simulink model "controlGPI_pos_3dof_conMI"  (R2023b)
settings: Solver=VariableStepAuto  StartTime=0.0  StopTime=tsim  FixedStep=1e-5  MaxStep=tstep  RelTol=1e-3
undefined symbols (not defined in the file): contr_robot_params, ddq, dq, MI_Contr1, MI_Contr2, MI_Contr3, MI_motor1, MI_motor2, MI_motor3, ndof, NN_Bspline_params, NN_RBF_params, nn_select, ns, Pc, q, q0, q_cero, q_eq, robot_params, sigbuilder_block, t_qeq_init, t_tr_init, t_trtr, tau_L, tau_L_mags, tr_muestra, Wc, Zc
libraries: mcbcontrolslib x6, spsRMSLib x6, simulink x2
(part 2 of 3)

== system controlGPI_pos_3dof_conMI/Actuadores (Motores de inducción)/MI1 + PBC Torque Controller/Calculo de Potencia eléctrica ==
  u_Sab : Inport
  i_Sab : Inport  Port=2
  Demux1 : Demux  Commented=on  Outputs=3
  Demux2 : Demux  Commented=on  Outputs=3
  Demux3 : Demux  Commented=on  Outputs=3
  Demux4 : Demux  Outputs=3
  From1 : From  Commented=on  GotoTag=u_S3abc
  From2 : From  Commented=on  GotoTag=i_S3abc
  IIR Filter : mcbcontrolslib/IIR Filter  Commented=on  VariantControl=Low Pass Filter  VariantSelect=Low-pass  Filter_constant=0.04  advancedSettings=on  Ts=50e-6  cutOff_freq=132.6291
      settings: LibrarySourceBlock=mcbhdllib/Signal Management/IIR Filter
  IIR Filter1 : mcbcontrolslib/IIR Filter  Commented=on  VariantControl=Low Pass Filter  VariantSelect=Low-pass  Filter_constant=0.04  advancedSettings=on  Ts=50e-6  cutOff_freq=132.6291
      settings: LibrarySourceBlock=mcbhdllib/Signal Management/IIR Filter
  Product1 : Product
  Product2 : Product  Commented=on
  RMS : spsRMSLib/RMS  Commented=on  TrueRMS=on  Freq=60  RMSInit=120  Ts=0
  RMS1 : spsRMSLib/RMS  Commented=on  TrueRMS=on  Freq=60  RMSInit=120  Ts=0
  Scope : Scope  Commented=on
  Scope1 : Scope  Commented=on
  Scope11 : Scope  Commented=on
  Sum1 : Sum  Inputs=|+++
  Sum2 : Sum  Commented=on  Inputs=|+++
  ab0 - ABC : MATLAB Function  TreatAsAtomicUnit=on
  ab0 - ABC1 : MATLAB Function  TreatAsAtomicUnit=on
  i_S3abc1 : Scope  Commented=on  NumInputPorts=3
  u_S3abc1 : Scope  Commented=on  NumInputPorts=3
  P_elect : Outport
  u_S3abc : Outport  Port=2
  i_S3abc : Outport  Port=3
  wires:
  Sum1/1 -> P_elect/1
  Demux4/1 -> Sum1/1
  [i_S3abc] -> Product1/2
  i_Sab/1 -> ab0 - ABC1/1(BPU)
  Demux4/3 -> Sum1/3
  [u_S3abc] -> Product1/1
  Demux4/2 -> Sum1/2
  Product1/1 -> Demux4/1
  u_Sab/1 -> ab0 - ABC/1(BPU)
  [u_S3abc] -> u_S3abc/1
  [i_S3abc] -> i_S3abc/1
  ab0 - ABC/1(U) -> [u_S3abc]
  ab0 - ABC1/1(U) -> [i_S3abc]
  IIR Filter/1 -> Product2/1, Demux1/1
  RMS/1 -> Scope11/1
  Demux1/2 -> u_S3abc1/2
  Demux1/3 -> u_S3abc1/3
  Demux1/1 -> RMS/1, u_S3abc1/1
  From1/1 -> IIR Filter/1
  Demux2/1 -> RMS1/1, i_S3abc1/1
  RMS1/1 -> Scope1/1
  Demux2/2 -> i_S3abc1/2
  IIR Filter1/1 -> Product2/2, Demux2/1
  From2/1 -> IIR Filter1/1
  Demux2/3 -> i_S3abc1/3
  Demux3/2 -> Sum2/2
  Demux3/3 -> Sum2/3
  Sum2/1 -> Scope/1
  Product2/1 -> Demux3/1
  Demux3/1 -> Sum2/1

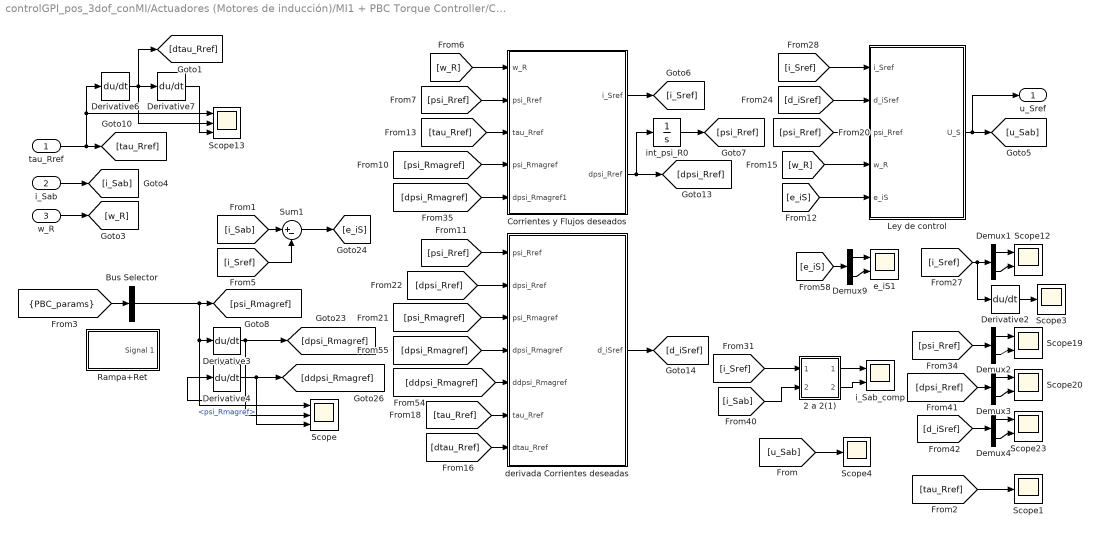
== system controlGPI_pos_3dof_conMI/Actuadores (Motores de inducción)/MI1 + PBC Torque Controller/Controlador PBC ==
  tau_Rref : Inport
  i_Sab : Inport  Port=2
  w_R : Inport  Port=3
  2 a 2(1) : Subsystem
  Bus Selector : BusSelector  OutputSignals=psi_Rmagref
  Corrientes y Flujos deseados : Subsystem
  Demux{1..4,9} (5 alike) : Demux  Outputs=2
  Derivative{2..4,6..7} (5 alike) : Derivative
  Ley de control : Subsystem
  Rampa+Ret : Subsystem  Tag=STV Subsys  LoadFcn=sigbuilder_block('load');  StartFcn=sigbuilder_block('start');  StopFcn=sigbuilder_block('stop');  ClipboardFcn=sigbuilder_block('clipboard');  mask(Sigbuilder block){tuvar=[0:10]}
      mask help: Sigbuilder GUI
      mask init:
      | if ~strcmp(get_param(bdroot(gcbh),'SimulationStatus'),'stopped') tuvar = sigbuilder_block('maskInit'); end
      settings: CopyFcn=sigbuilder_block('copy');  DeleteFcn=sigbuilder_block('delete');  ModelCloseFcn=sigbuilder_block('modelClose');  PreSaveFcn=sigbuilder_block('preSave');  PauseFcn=sigbuilder_block('pause')  ContinueFcn=sigbuilder_block('continue')  NameChangeFcn=sigbuilder_block('namechange');  OpenFcn=sigbuilder_block('open',[280.5 86.5 550.5 399.5 ]);  CloseFcn=sigbuilder_block('close');
      mask Display: plot(0, 0, 100, 100,[2, 2, 32, 32, 2], [68, 8, 8, 68, 68],[32, 2], [38, 38], [32, 19, 2],[53, 60, 44], [32, 17, 17, 2],[16, 16, 31, 31]);txt = getActiveGroup(gcbh);text(2, 100, txt,'verticalAlignment', 'top');
  Scope : Scope  NumInputPorts=3
  Scope1 : Scope
  Scope{12,19..20,23} (4 alike) : Scope  NumInputPorts=2
  Scope13 : Scope  NumInputPorts=3
  Scope3 : Scope
  Scope4 : Scope
  Sum1 : Sum  Inputs=|+-
  derivada Corrientes deseadas : Subsystem
  e_iS1 : Scope  NumInputPorts=2
  i_Sab_comp : Scope  NumInputPorts=2
  int_psi_R0 : Integrator  InitialCondition=[0.51032;0]
  u_Sref : Outport
  wires:
  Derivative3/1 -> Scope/2, Derivative4/1, [dpsi_Rmagref]
  Derivative4/1 -> [ddpsi_Rmagref], Scope/3
  Bus Selector/1 -> Scope/1, Derivative3/1, [psi_Rmagref]  "<psi_Rmagref>"
  i_Sab/1 -> [i_Sab]
  Demux1/1 -> Scope12/1
  [d_iSref] -> Demux4/1
  Demux3/2 -> Scope20/2
  Demux2/1 -> Scope19/1
  Demux1/2 -> Scope12/2
  [dpsi_Rref] -> Demux3/1
  Demux3/1 -> Scope20/1
  Demux4/1 -> Scope23/1
  [psi_Rref] -> Demux2/1
  Demux4/2 -> Scope23/2
  Demux2/2 -> Scope19/2
  [tau_Rref] -> Corrientes y Flujos deseados/3(tau_Rref)
  [w_R] -> Corrientes y Flujos deseados/1(w_R)
  int_psi_R0/1 -> [psi_Rref]
  Corrientes y Flujos deseados/2(dpsi_Rref) -> int_psi_R0/1, [dpsi_Rref]
  [psi_Rref] -> Corrientes y Flujos deseados/2(psi_Rref)
  [psi_Rmagref] -> Corrientes y Flujos deseados/4(psi_Rmagref)
  [dpsi_Rmagref] -> Corrientes y Flujos deseados/5(dpsi_Rmagref1)
  [psi_Rref] -> derivada Corrientes deseadas/1(psi_Rref)
  [dpsi_Rref] -> derivada Corrientes deseadas/2(dpsi_Rref)
  [psi_Rmagref] -> derivada Corrientes deseadas/3(psi_Rmagref)
  [dpsi_Rmagref] -> derivada Corrientes deseadas/4(dpsi_Rmagref)
  [ddpsi_Rmagref] -> derivada Corrientes deseadas/5(ddpsi_Rmagref)
  [tau_Rref] -> derivada Corrientes deseadas/6(tau_Rref)
  [dtau_Rref] -> derivada Corrientes deseadas/7(dtau_Rref)
  derivada Corrientes deseadas/1(d_iSref) -> [d_iSref]
  [e_iS] -> Demux9/1
  Demux9/1 -> e_iS1/1
  Demux9/2 -> e_iS1/2
  [i_Sab] -> Sum1/1
  [i_Sref] -> Sum1/2
  Sum1/1 -> [e_iS]
  [u_Sab] -> Scope4/1
  [i_Sref] -> Ley de control/1(i_Sref)
  [d_iSref] -> Ley de control/2(d_iSref)
  [psi_Rref] -> Ley de control/3(psi_Rref)
  [w_R] -> Ley de control/4(w_R)
  Ley de control/1(U_S) -> u_Sref/1, [u_Sab]
  [e_iS] -> Ley de control/5(e_iS)
  Derivative7/1 -> Scope13/3
  tau_Rref/1 -> Derivative6/1, Scope13/1, [tau_Rref]
  Derivative6/1 -> [dtau_Rref], Derivative7/1, Scope13/2
  2 a 2(1)/2(Out2) -> i_Sab_comp/2
  2 a 2(1)/1(Out1) -> i_Sab_comp/1
  [i_Sab] -> 2 a 2(1)/2(In2)
  [i_Sref] -> 2 a 2(1)/1(In1)
  [i_Sref] -> Derivative2/1, Demux1/1
  Derivative2/1 -> Scope3/1
  w_R/1 -> [w_R]
  [tau_Rref] -> Scope1/1
  [PBC_params] -> Bus Selector/1
  Corrientes y Flujos deseados/1(i_Sref) -> [i_Sref]

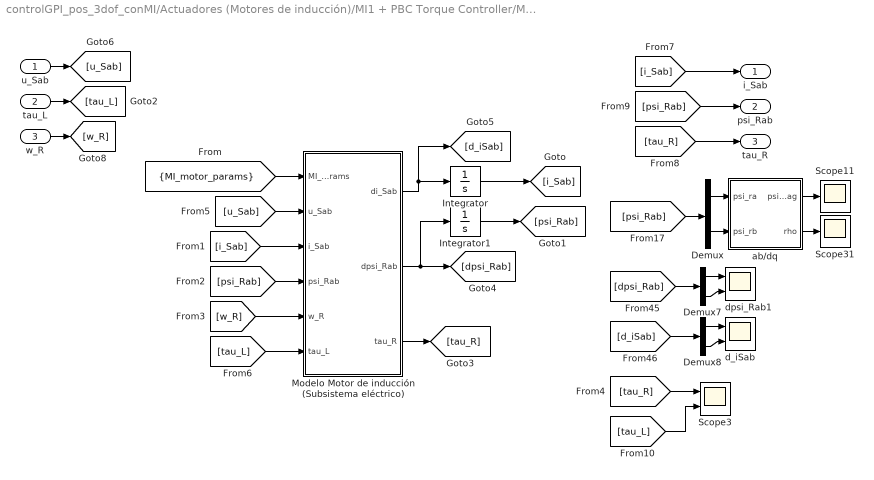
== system controlGPI_pos_3dof_conMI/Actuadores (Motores de inducción)/MI1 + PBC Torque Controller/Modelo MI (Subsistema eléctrico) ==
  u_Sab : Inport
  tau_L : Inport  Port=2
  w_R : Inport  Port=3
  Demux : Demux  Outputs=2
  Demux7 : Demux  Outputs=2
  Demux8 : Demux  Outputs=2
  Integrator : Integrator
  Integrator1 : Integrator
  Modelo Motor de inducción (Subsistema eléctrico) : MATLAB Function  TreatAsAtomicUnit=on
  Scope11 : Scope
  Scope3 : Scope  NumInputPorts=2
  Scope31 : Scope
  ab/dq : MATLAB Function  TreatAsAtomicUnit=on
  d_iSab : Scope  NumInputPorts=2
  dpsi_Rab1 : Scope  NumInputPorts=2
  i_Sab : Outport
  psi_Rab : Outport  Port=2
  tau_R : Outport  Port=3
  wires:
  Modelo Motor de inducción (Subsistema eléctrico)/1(di_Sab) -> Integrator/1, [d_iSab]
  Modelo Motor de inducción (Subsistema eléctrico)/2(dpsi_Rab) -> Integrator1/1, [dpsi_Rab]
  [w_R] -> Modelo Motor de inducción (Subsistema eléctrico)/5(w_R)
  [psi_Rab] -> Modelo Motor de inducción (Subsistema eléctrico)/4(psi_Rab)
  [i_Sab] -> Modelo Motor de inducción (Subsistema eléctrico)/3(i_Sab)
  Integrator1/1 -> [psi_Rab]
  u_Sab/1 -> [u_Sab]
  Modelo Motor de inducción (Subsistema eléctrico)/3(tau_R) -> [tau_R]
  [tau_R] -> Scope3/1
  ab/dq/1(psi_Rmag) -> Scope11/1
  [psi_Rab] -> Demux/1
  Demux7/1 -> dpsi_Rab1/1
  Demux7/2 -> dpsi_Rab1/2
  [d_iSab] -> Demux8/1
  ab/dq/2(rho) -> Scope31/1
  Demux/1 -> ab/dq/1(psi_ra)
  Demux8/2 -> d_iSab/2
  Demux8/1 -> d_iSab/1
  [dpsi_Rab] -> Demux7/1
  Demux/2 -> ab/dq/2(psi_rb)
  Integrator/1 -> [i_Sab]
  [MI_motor_params] -> Modelo Motor de inducción (Subsistema eléctrico)/1(MI_motor_params)
  [u_Sab] -> Modelo Motor de inducción (Subsistema eléctrico)/2(u_Sab)
  tau_L/1 -> [tau_L]
  [tau_L] -> Modelo Motor de inducción (Subsistema eléctrico)/6(tau_L)
  w_R/1 -> [w_R]
  [tau_R] -> tau_R/1
  [psi_Rab] -> psi_Rab/1
  [i_Sab] -> i_Sab/1
  [tau_L] -> Scope3/2

== system controlGPI_pos_3dof_conMI/Actuadores (Motores de inducción)/MI2 + PBC Torque Controller/Calculo de Potencia eléctrica ==
  u_Sab : Inport
  i_Sab : Inport  Port=2
  Demux1 : Demux  Commented=on  Outputs=3
  Demux2 : Demux  Commented=on  Outputs=3
  Demux3 : Demux  Commented=on  Outputs=3
  Demux4 : Demux  Outputs=3
  From1 : From  Commented=on  GotoTag=u_S3abc
  From2 : From  Commented=on  GotoTag=i_S3abc
  IIR Filter : mcbcontrolslib/IIR Filter  Commented=on  VariantControl=Low Pass Filter  VariantSelect=Low-pass  Filter_constant=0.04  advancedSettings=on  Ts=50e-6  cutOff_freq=132.6291
      settings: LibrarySourceBlock=mcbhdllib/Signal Management/IIR Filter
  IIR Filter1 : mcbcontrolslib/IIR Filter  Commented=on  VariantControl=Low Pass Filter  VariantSelect=Low-pass  Filter_constant=0.04  advancedSettings=on  Ts=50e-6  cutOff_freq=132.6291
      settings: LibrarySourceBlock=mcbhdllib/Signal Management/IIR Filter
  Product1 : Product
  Product2 : Product  Commented=on
  RMS : spsRMSLib/RMS  Commented=on  TrueRMS=on  Freq=60  RMSInit=120  Ts=0
  RMS1 : spsRMSLib/RMS  Commented=on  TrueRMS=on  Freq=60  RMSInit=120  Ts=0
  Scope : Scope  Commented=on
  Scope1 : Scope  Commented=on
  Scope11 : Scope  Commented=on
  Sum1 : Sum  Inputs=|+++
  Sum2 : Sum  Commented=on  Inputs=|+++
  ab0 - ABC : MATLAB Function  TreatAsAtomicUnit=on
  ab0 - ABC1 : MATLAB Function  TreatAsAtomicUnit=on
  i_S3abc1 : Scope  Commented=on  NumInputPorts=3
  u_S3abc1 : Scope  Commented=on  NumInputPorts=3
  P_elect : Outport
  u_S3abc : Outport  Port=2
  i_S3abc : Outport  Port=3
  wires:
  Sum1/1 -> P_elect/1
  Demux4/1 -> Sum1/1
  [i_S3abc] -> Product1/2
  i_Sab/1 -> ab0 - ABC1/1(BPU)
  Demux4/3 -> Sum1/3
  [u_S3abc] -> Product1/1
  Demux4/2 -> Sum1/2
  Product1/1 -> Demux4/1
  u_Sab/1 -> ab0 - ABC/1(BPU)
  [u_S3abc] -> u_S3abc/1
  [i_S3abc] -> i_S3abc/1
  ab0 - ABC/1(U) -> [u_S3abc]
  ab0 - ABC1/1(U) -> [i_S3abc]
  IIR Filter/1 -> Product2/1, Demux1/1
  RMS/1 -> Scope11/1
  Demux1/2 -> u_S3abc1/2
  Demux1/3 -> u_S3abc1/3
  Demux1/1 -> RMS/1, u_S3abc1/1
  From1/1 -> IIR Filter/1
  Demux2/1 -> RMS1/1, i_S3abc1/1
  RMS1/1 -> Scope1/1
  Demux2/2 -> i_S3abc1/2
  IIR Filter1/1 -> Product2/2, Demux2/1
  From2/1 -> IIR Filter1/1
  Demux2/3 -> i_S3abc1/3
  Demux3/2 -> Sum2/2
  Demux3/3 -> Sum2/3
  Sum2/1 -> Scope/1
  Product2/1 -> Demux3/1
  Demux3/1 -> Sum2/1

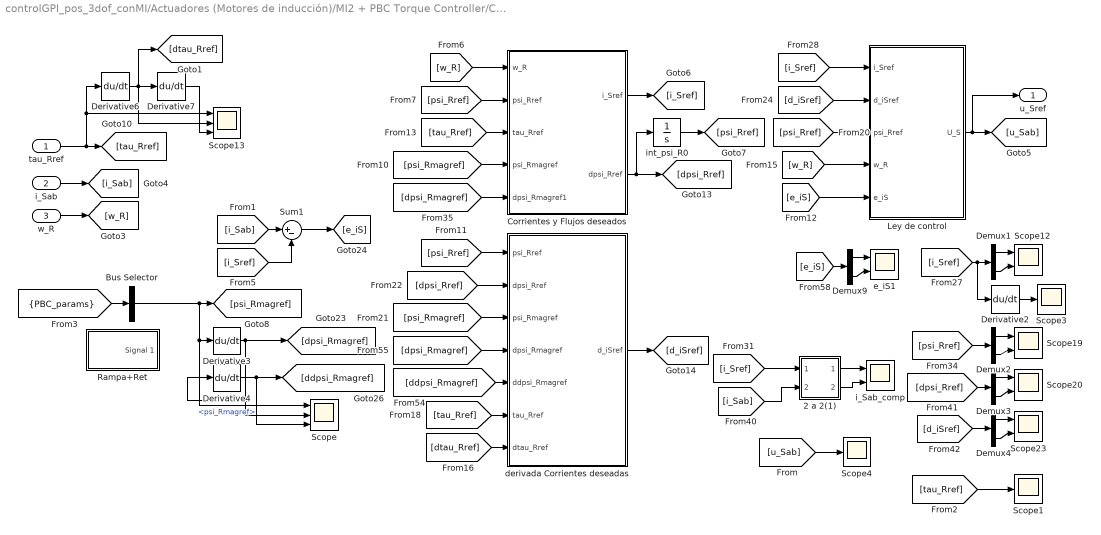
== system controlGPI_pos_3dof_conMI/Actuadores (Motores de inducción)/MI2 + PBC Torque Controller/Controlador PBC ==
  tau_Rref : Inport
  i_Sab : Inport  Port=2
  w_R : Inport  Port=3
  2 a 2(1) : Subsystem
  Bus Selector : BusSelector  OutputSignals=psi_Rmagref
  Corrientes y Flujos deseados : Subsystem
  Demux{1..4,9} (5 alike) : Demux  Outputs=2
  Derivative{2..4,6..7} (5 alike) : Derivative
  Ley de control : Subsystem
  Rampa+Ret : Subsystem  Tag=STV Subsys  LoadFcn=sigbuilder_block('load');  StartFcn=sigbuilder_block('start');  StopFcn=sigbuilder_block('stop');  ClipboardFcn=sigbuilder_block('clipboard');  mask(Sigbuilder block){tuvar=[0:10]}
      mask help: Sigbuilder GUI
      mask init:
      | if ~strcmp(get_param(bdroot(gcbh),'SimulationStatus'),'stopped') tuvar = sigbuilder_block('maskInit'); end
      settings: CopyFcn=sigbuilder_block('copy');  DeleteFcn=sigbuilder_block('delete');  ModelCloseFcn=sigbuilder_block('modelClose');  PreSaveFcn=sigbuilder_block('preSave');  PauseFcn=sigbuilder_block('pause')  ContinueFcn=sigbuilder_block('continue')  NameChangeFcn=sigbuilder_block('namechange');  OpenFcn=sigbuilder_block('open',[280.5 86.5 550.5 399.5 ]);  CloseFcn=sigbuilder_block('close');
      mask Display: plot(0, 0, 100, 100,[2, 2, 32, 32, 2], [68, 8, 8, 68, 68],[32, 2], [38, 38], [32, 19, 2],[53, 60, 44], [32, 17, 17, 2],[16, 16, 31, 31]);txt = getActiveGroup(gcbh);text(2, 100, txt,'verticalAlignment', 'top');
  Scope : Scope  NumInputPorts=3
  Scope1 : Scope
  Scope{12,19..20,23} (4 alike) : Scope  NumInputPorts=2
  Scope13 : Scope  NumInputPorts=3
  Scope3 : Scope
  Scope4 : Scope
  Sum1 : Sum  Inputs=|+-
  derivada Corrientes deseadas : Subsystem
  e_iS1 : Scope  NumInputPorts=2
  i_Sab_comp : Scope  NumInputPorts=2
  int_psi_R0 : Integrator  InitialCondition=[0.51032;0]
  u_Sref : Outport
  wires:
  Derivative3/1 -> Scope/2, Derivative4/1, [dpsi_Rmagref]
  Derivative4/1 -> [ddpsi_Rmagref], Scope/3
  Bus Selector/1 -> Scope/1, Derivative3/1, [psi_Rmagref]  "<psi_Rmagref>"
  i_Sab/1 -> [i_Sab]
  Demux1/1 -> Scope12/1
  [d_iSref] -> Demux4/1
  Demux3/2 -> Scope20/2
  Demux2/1 -> Scope19/1
  Demux1/2 -> Scope12/2
  [dpsi_Rref] -> Demux3/1
  Demux3/1 -> Scope20/1
  Demux4/1 -> Scope23/1
  [psi_Rref] -> Demux2/1
  Demux4/2 -> Scope23/2
  Demux2/2 -> Scope19/2
  [tau_Rref] -> Corrientes y Flujos deseados/3(tau_Rref)
  [w_R] -> Corrientes y Flujos deseados/1(w_R)
  int_psi_R0/1 -> [psi_Rref]
  Corrientes y Flujos deseados/2(dpsi_Rref) -> int_psi_R0/1, [dpsi_Rref]
  [psi_Rref] -> Corrientes y Flujos deseados/2(psi_Rref)
  [psi_Rmagref] -> Corrientes y Flujos deseados/4(psi_Rmagref)
  [dpsi_Rmagref] -> Corrientes y Flujos deseados/5(dpsi_Rmagref1)
  [psi_Rref] -> derivada Corrientes deseadas/1(psi_Rref)
  [dpsi_Rref] -> derivada Corrientes deseadas/2(dpsi_Rref)
  [psi_Rmagref] -> derivada Corrientes deseadas/3(psi_Rmagref)
  [dpsi_Rmagref] -> derivada Corrientes deseadas/4(dpsi_Rmagref)
  [ddpsi_Rmagref] -> derivada Corrientes deseadas/5(ddpsi_Rmagref)
  [tau_Rref] -> derivada Corrientes deseadas/6(tau_Rref)
  [dtau_Rref] -> derivada Corrientes deseadas/7(dtau_Rref)
  derivada Corrientes deseadas/1(d_iSref) -> [d_iSref]
  [e_iS] -> Demux9/1
  Demux9/1 -> e_iS1/1
  Demux9/2 -> e_iS1/2
  [i_Sab] -> Sum1/1
  [i_Sref] -> Sum1/2
  Sum1/1 -> [e_iS]
  [u_Sab] -> Scope4/1
  [i_Sref] -> Ley de control/1(i_Sref)
  [d_iSref] -> Ley de control/2(d_iSref)
  [psi_Rref] -> Ley de control/3(psi_Rref)
  [w_R] -> Ley de control/4(w_R)
  Ley de control/1(U_S) -> u_Sref/1, [u_Sab]
  [e_iS] -> Ley de control/5(e_iS)
  Derivative7/1 -> Scope13/3
  tau_Rref/1 -> Derivative6/1, Scope13/1, [tau_Rref]
  Derivative6/1 -> [dtau_Rref], Derivative7/1, Scope13/2
  2 a 2(1)/2(Out2) -> i_Sab_comp/2
  2 a 2(1)/1(Out1) -> i_Sab_comp/1
  [i_Sab] -> 2 a 2(1)/2(In2)
  [i_Sref] -> 2 a 2(1)/1(In1)
  [i_Sref] -> Derivative2/1, Demux1/1
  Derivative2/1 -> Scope3/1
  w_R/1 -> [w_R]
  [tau_Rref] -> Scope1/1
  [PBC_params] -> Bus Selector/1
  Corrientes y Flujos deseados/1(i_Sref) -> [i_Sref]

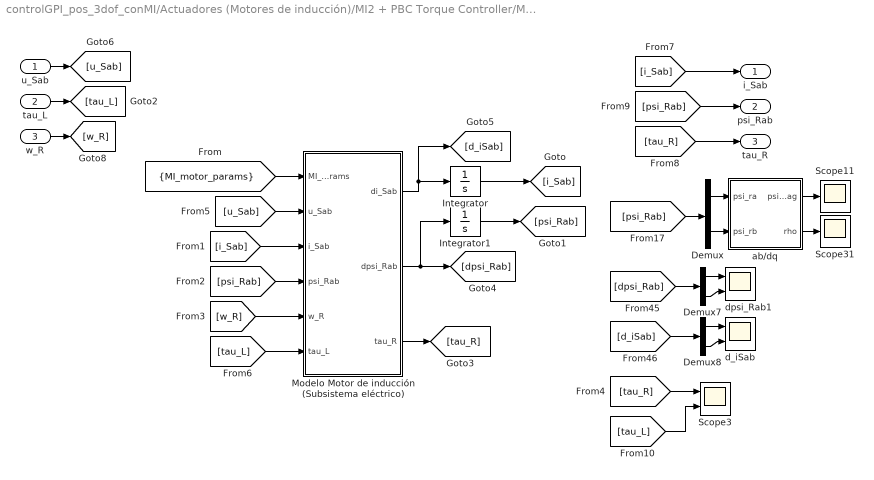
== system controlGPI_pos_3dof_conMI/Actuadores (Motores de inducción)/MI2 + PBC Torque Controller/Modelo MI (Subsistema eléctrico) ==
  u_Sab : Inport
  tau_L : Inport  Port=2
  w_R : Inport  Port=3
  Demux : Demux  Outputs=2
  Demux7 : Demux  Outputs=2
  Demux8 : Demux  Outputs=2
  Integrator : Integrator
  Integrator1 : Integrator
  Modelo Motor de inducción (Subsistema eléctrico) : MATLAB Function  TreatAsAtomicUnit=on
  Scope11 : Scope
  Scope3 : Scope  NumInputPorts=2
  Scope31 : Scope
  ab/dq : MATLAB Function  TreatAsAtomicUnit=on
  d_iSab : Scope  NumInputPorts=2
  dpsi_Rab1 : Scope  NumInputPorts=2
  i_Sab : Outport
  psi_Rab : Outport  Port=2
  tau_R : Outport  Port=3
  wires:
  Modelo Motor de inducción (Subsistema eléctrico)/1(di_Sab) -> Integrator/1, [d_iSab]
  Modelo Motor de inducción (Subsistema eléctrico)/2(dpsi_Rab) -> Integrator1/1, [dpsi_Rab]
  [w_R] -> Modelo Motor de inducción (Subsistema eléctrico)/5(w_R)
  [psi_Rab] -> Modelo Motor de inducción (Subsistema eléctrico)/4(psi_Rab)
  [i_Sab] -> Modelo Motor de inducción (Subsistema eléctrico)/3(i_Sab)
  Integrator1/1 -> [psi_Rab]
  u_Sab/1 -> [u_Sab]
  Modelo Motor de inducción (Subsistema eléctrico)/3(tau_R) -> [tau_R]
  [tau_R] -> Scope3/1
  ab/dq/1(psi_Rmag) -> Scope11/1
  [psi_Rab] -> Demux/1
  Demux7/1 -> dpsi_Rab1/1
  Demux7/2 -> dpsi_Rab1/2
  [d_iSab] -> Demux8/1
  ab/dq/2(rho) -> Scope31/1
  Demux/1 -> ab/dq/1(psi_ra)
  Demux8/2 -> d_iSab/2
  Demux8/1 -> d_iSab/1
  [dpsi_Rab] -> Demux7/1
  Demux/2 -> ab/dq/2(psi_rb)
  Integrator/1 -> [i_Sab]
  [MI_motor_params] -> Modelo Motor de inducción (Subsistema eléctrico)/1(MI_motor_params)
  [u_Sab] -> Modelo Motor de inducción (Subsistema eléctrico)/2(u_Sab)
  tau_L/1 -> [tau_L]
  [tau_L] -> Modelo Motor de inducción (Subsistema eléctrico)/6(tau_L)
  w_R/1 -> [w_R]
  [tau_R] -> tau_R/1
  [psi_Rab] -> psi_Rab/1
  [i_Sab] -> i_Sab/1
  [tau_L] -> Scope3/2

== system controlGPI_pos_3dof_conMI/Actuadores (Motores de inducción)/MI3 + PBC Torque Controller/Calculo de Potencia eléctrica ==
  u_Sab : Inport
  i_Sab : Inport  Port=2
  Demux1 : Demux  Commented=on  Outputs=3
  Demux2 : Demux  Commented=on  Outputs=3
  Demux3 : Demux  Commented=on  Outputs=3
  Demux4 : Demux  Outputs=3
  From1 : From  Commented=on  GotoTag=u_S3abc
  From2 : From  Commented=on  GotoTag=i_S3abc
  IIR Filter : mcbcontrolslib/IIR Filter  Commented=on  VariantControl=Low Pass Filter  VariantSelect=Low-pass  Filter_constant=0.04  advancedSettings=on  Ts=50e-6  cutOff_freq=132.6291
      settings: LibrarySourceBlock=mcbhdllib/Signal Management/IIR Filter
  IIR Filter1 : mcbcontrolslib/IIR Filter  Commented=on  VariantControl=Low Pass Filter  VariantSelect=Low-pass  Filter_constant=0.04  advancedSettings=on  Ts=50e-6  cutOff_freq=132.6291
      settings: LibrarySourceBlock=mcbhdllib/Signal Management/IIR Filter
  Product1 : Product
  Product2 : Product  Commented=on
  RMS : spsRMSLib/RMS  Commented=on  TrueRMS=on  Freq=60  RMSInit=120  Ts=0
  RMS1 : spsRMSLib/RMS  Commented=on  TrueRMS=on  Freq=60  RMSInit=120  Ts=0
  Scope : Scope  Commented=on
  Scope1 : Scope  Commented=on
  Scope11 : Scope  Commented=on
  Sum1 : Sum  Inputs=|+++
  Sum2 : Sum  Commented=on  Inputs=|+++
  ab0 - ABC : MATLAB Function  TreatAsAtomicUnit=on
  ab0 - ABC1 : MATLAB Function  TreatAsAtomicUnit=on
  i_S3abc1 : Scope  Commented=on  NumInputPorts=3
  u_S3abc1 : Scope  Commented=on  NumInputPorts=3
  P_elect : Outport
  u_S3abc : Outport  Port=2
  i_S3abc : Outport  Port=3
  wires:
  Sum1/1 -> P_elect/1
  Demux4/1 -> Sum1/1
  [i_S3abc] -> Product1/2
  i_Sab/1 -> ab0 - ABC1/1(BPU)
  Demux4/3 -> Sum1/3
  [u_S3abc] -> Product1/1
  Demux4/2 -> Sum1/2
  Product1/1 -> Demux4/1
  u_Sab/1 -> ab0 - ABC/1(BPU)
  [u_S3abc] -> u_S3abc/1
  [i_S3abc] -> i_S3abc/1
  ab0 - ABC/1(U) -> [u_S3abc]
  ab0 - ABC1/1(U) -> [i_S3abc]
  IIR Filter/1 -> Product2/1, Demux1/1
  RMS/1 -> Scope11/1
  Demux1/2 -> u_S3abc1/2
  Demux1/3 -> u_S3abc1/3
  Demux1/1 -> RMS/1, u_S3abc1/1
  From1/1 -> IIR Filter/1
  Demux2/1 -> RMS1/1, i_S3abc1/1
  RMS1/1 -> Scope1/1
  Demux2/2 -> i_S3abc1/2
  IIR Filter1/1 -> Product2/2, Demux2/1
  From2/1 -> IIR Filter1/1
  Demux2/3 -> i_S3abc1/3
  Demux3/2 -> Sum2/2
  Demux3/3 -> Sum2/3
  Sum2/1 -> Scope/1
  Product2/1 -> Demux3/1
  Demux3/1 -> Sum2/1

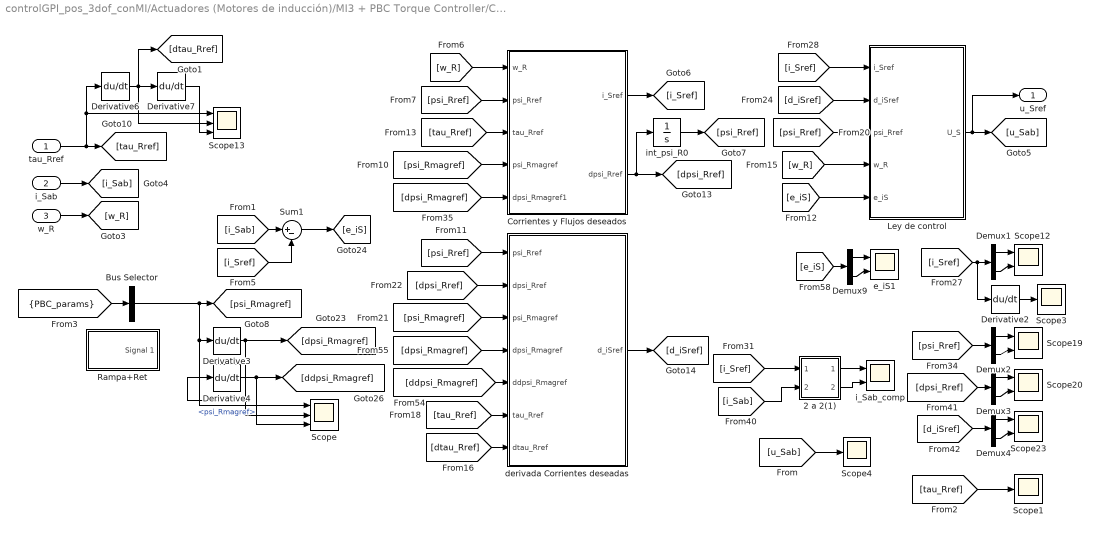
== system controlGPI_pos_3dof_conMI/Actuadores (Motores de inducción)/MI3 + PBC Torque Controller/Controlador PBC ==
  tau_Rref : Inport
  i_Sab : Inport  Port=2
  w_R : Inport  Port=3
  2 a 2(1) : Subsystem
  Bus Selector : BusSelector  OutputSignals=psi_Rmagref
  Corrientes y Flujos deseados : Subsystem
  Demux{1..4,9} (5 alike) : Demux  Outputs=2
  Derivative{2..4,6..7} (5 alike) : Derivative
  Ley de control : Subsystem
  Rampa+Ret : Subsystem  Tag=STV Subsys  LoadFcn=sigbuilder_block('load');  StartFcn=sigbuilder_block('start');  StopFcn=sigbuilder_block('stop');  ClipboardFcn=sigbuilder_block('clipboard');  mask(Sigbuilder block){tuvar=[0:10]}
      mask help: Sigbuilder GUI
      mask init:
      | if ~strcmp(get_param(bdroot(gcbh),'SimulationStatus'),'stopped') tuvar = sigbuilder_block('maskInit'); end
      settings: CopyFcn=sigbuilder_block('copy');  DeleteFcn=sigbuilder_block('delete');  ModelCloseFcn=sigbuilder_block('modelClose');  PreSaveFcn=sigbuilder_block('preSave');  PauseFcn=sigbuilder_block('pause')  ContinueFcn=sigbuilder_block('continue')  NameChangeFcn=sigbuilder_block('namechange');  OpenFcn=sigbuilder_block('open',[280.5 86.5 550.5 399.5 ]);  CloseFcn=sigbuilder_block('close');
      mask Display: plot(0, 0, 100, 100,[2, 2, 32, 32, 2], [68, 8, 8, 68, 68],[32, 2], [38, 38], [32, 19, 2],[53, 60, 44], [32, 17, 17, 2],[16, 16, 31, 31]);txt = getActiveGroup(gcbh);text(2, 100, txt,'verticalAlignment', 'top');
  Scope : Scope  NumInputPorts=3
  Scope1 : Scope
  Scope{12,19..20,23} (4 alike) : Scope  NumInputPorts=2
  Scope13 : Scope  NumInputPorts=3
  Scope3 : Scope
  Scope4 : Scope
  Sum1 : Sum  Inputs=|+-
  derivada Corrientes deseadas : Subsystem
  e_iS1 : Scope  NumInputPorts=2
  i_Sab_comp : Scope  NumInputPorts=2
  int_psi_R0 : Integrator  InitialCondition=[0.51032;0]
  u_Sref : Outport
  wires:
  Derivative3/1 -> Scope/2, Derivative4/1, [dpsi_Rmagref]
  Derivative4/1 -> [ddpsi_Rmagref], Scope/3
  Bus Selector/1 -> Scope/1, Derivative3/1, [psi_Rmagref]  "<psi_Rmagref>"
  i_Sab/1 -> [i_Sab]
  Demux1/1 -> Scope12/1
  [d_iSref] -> Demux4/1
  Demux3/2 -> Scope20/2
  Demux2/1 -> Scope19/1
  Demux1/2 -> Scope12/2
  [dpsi_Rref] -> Demux3/1
  Demux3/1 -> Scope20/1
  Demux4/1 -> Scope23/1
  [psi_Rref] -> Demux2/1
  Demux4/2 -> Scope23/2
  Demux2/2 -> Scope19/2
  [tau_Rref] -> Corrientes y Flujos deseados/3(tau_Rref)
  [w_R] -> Corrientes y Flujos deseados/1(w_R)
  int_psi_R0/1 -> [psi_Rref]
  Corrientes y Flujos deseados/2(dpsi_Rref) -> int_psi_R0/1, [dpsi_Rref]
  [psi_Rref] -> Corrientes y Flujos deseados/2(psi_Rref)
  [psi_Rmagref] -> Corrientes y Flujos deseados/4(psi_Rmagref)
  [dpsi_Rmagref] -> Corrientes y Flujos deseados/5(dpsi_Rmagref1)
  [psi_Rref] -> derivada Corrientes deseadas/1(psi_Rref)
  [dpsi_Rref] -> derivada Corrientes deseadas/2(dpsi_Rref)
  [psi_Rmagref] -> derivada Corrientes deseadas/3(psi_Rmagref)
  [dpsi_Rmagref] -> derivada Corrientes deseadas/4(dpsi_Rmagref)
  [ddpsi_Rmagref] -> derivada Corrientes deseadas/5(ddpsi_Rmagref)
  [tau_Rref] -> derivada Corrientes deseadas/6(tau_Rref)
  [dtau_Rref] -> derivada Corrientes deseadas/7(dtau_Rref)
  derivada Corrientes deseadas/1(d_iSref) -> [d_iSref]
  [e_iS] -> Demux9/1
  Demux9/1 -> e_iS1/1
  Demux9/2 -> e_iS1/2
  [i_Sab] -> Sum1/1
  [i_Sref] -> Sum1/2
  Sum1/1 -> [e_iS]
  [u_Sab] -> Scope4/1
  [i_Sref] -> Ley de control/1(i_Sref)
  [d_iSref] -> Ley de control/2(d_iSref)
  [psi_Rref] -> Ley de control/3(psi_Rref)
  [w_R] -> Ley de control/4(w_R)
  Ley de control/1(U_S) -> u_Sref/1, [u_Sab]
  [e_iS] -> Ley de control/5(e_iS)
  Derivative7/1 -> Scope13/3
  tau_Rref/1 -> Derivative6/1, Scope13/1, [tau_Rref]
  Derivative6/1 -> [dtau_Rref], Derivative7/1, Scope13/2
  2 a 2(1)/2(Out2) -> i_Sab_comp/2
  2 a 2(1)/1(Out1) -> i_Sab_comp/1
  [i_Sab] -> 2 a 2(1)/2(In2)
  [i_Sref] -> 2 a 2(1)/1(In1)
  [i_Sref] -> Derivative2/1, Demux1/1
  Derivative2/1 -> Scope3/1
  w_R/1 -> [w_R]
  [tau_Rref] -> Scope1/1
  [PBC_params] -> Bus Selector/1
  Corrientes y Flujos deseados/1(i_Sref) -> [i_Sref]

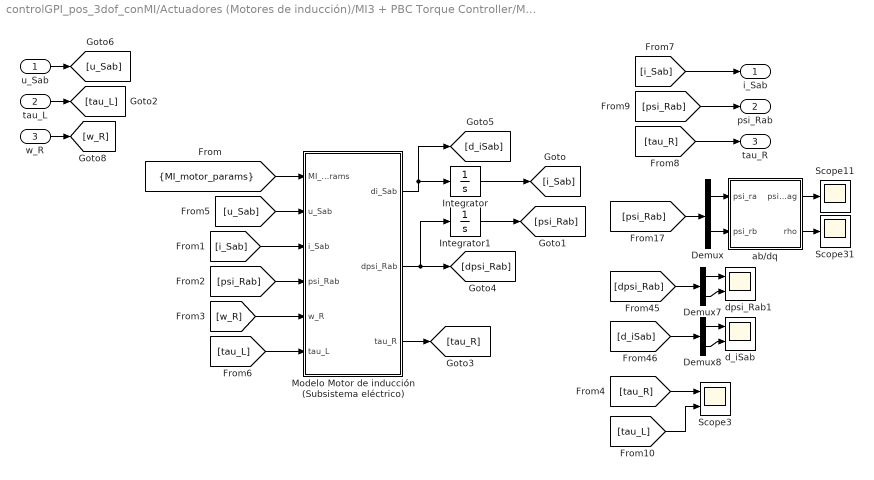
== system controlGPI_pos_3dof_conMI/Actuadores (Motores de inducción)/MI3 + PBC Torque Controller/Modelo MI (Subsistema eléctrico) ==
  u_Sab : Inport
  tau_L : Inport  Port=2
  w_R : Inport  Port=3
  Demux : Demux  Outputs=2
  Demux7 : Demux  Outputs=2
  Demux8 : Demux  Outputs=2
  Integrator : Integrator
  Integrator1 : Integrator
  Modelo Motor de inducción (Subsistema eléctrico) : MATLAB Function  TreatAsAtomicUnit=on
  Scope11 : Scope
  Scope3 : Scope  NumInputPorts=2
  Scope31 : Scope
  ab/dq : MATLAB Function  TreatAsAtomicUnit=on
  d_iSab : Scope  NumInputPorts=2
  dpsi_Rab1 : Scope  NumInputPorts=2
  i_Sab : Outport
  psi_Rab : Outport  Port=2
  tau_R : Outport  Port=3
  wires:
  Modelo Motor de inducción (Subsistema eléctrico)/1(di_Sab) -> Integrator/1, [d_iSab]
  Modelo Motor de inducción (Subsistema eléctrico)/2(dpsi_Rab) -> Integrator1/1, [dpsi_Rab]
  [w_R] -> Modelo Motor de inducción (Subsistema eléctrico)/5(w_R)
  [psi_Rab] -> Modelo Motor de inducción (Subsistema eléctrico)/4(psi_Rab)
  [i_Sab] -> Modelo Motor de inducción (Subsistema eléctrico)/3(i_Sab)
  Integrator1/1 -> [psi_Rab]
  u_Sab/1 -> [u_Sab]
  Modelo Motor de inducción (Subsistema eléctrico)/3(tau_R) -> [tau_R]
  [tau_R] -> Scope3/1
  ab/dq/1(psi_Rmag) -> Scope11/1
  [psi_Rab] -> Demux/1
  Demux7/1 -> dpsi_Rab1/1
  Demux7/2 -> dpsi_Rab1/2
  [d_iSab] -> Demux8/1
  ab/dq/2(rho) -> Scope31/1
  Demux/1 -> ab/dq/1(psi_ra)
  Demux8/2 -> d_iSab/2
  Demux8/1 -> d_iSab/1
  [dpsi_Rab] -> Demux7/1
  Demux/2 -> ab/dq/2(psi_rb)
  Integrator/1 -> [i_Sab]
  [MI_motor_params] -> Modelo Motor de inducción (Subsistema eléctrico)/1(MI_motor_params)
  [u_Sab] -> Modelo Motor de inducción (Subsistema eléctrico)/2(u_Sab)
  tau_L/1 -> [tau_L]
  [tau_L] -> Modelo Motor de inducción (Subsistema eléctrico)/6(tau_L)
  w_R/1 -> [w_R]
  [tau_R] -> tau_R/1
  [psi_Rab] -> psi_Rab/1
  [i_Sab] -> i_Sab/1
  [tau_L] -> Scope3/2

== system controlGPI_pos_3dof_conMI/ControladorGPI + NN/Red neuronal/B-Spline NNs ==
  e_q : Inport
  de_q : Inport  Port=2
  e_p : Inport  Port=3
  Action Port : ActionPort  ActionPortLabel=if(u1 == 1)
  Bus Creator : BusCreator  Inputs=3
  Constant3 : Constant  Value=NN_Bspline_params.struct  OutDataTypeStr=Bus: NN_Bspline_params_bus
  Data Store Memory : DataStoreMemory  DataStoreName=weightsWc  WriteAfterWriteMsg=warning  InitialValue=NN_Bspline_params.weights.weightWc  ShowAdditionalParam=off  OutDataTypeStr=double
  Data Store Memory1 : DataStoreMemory  DataStoreName=weightsZc  WriteAfterWriteMsg=warning  InitialValue=NN_Bspline_params.weights.weightZc  ShowAdditionalParam=off  OutDataTypeStr=double
  Data Store Memory2 : DataStoreMemory  DataStoreName=weightsPc  WriteAfterWriteMsg=warning  InitialValue=NN_Bspline_params.weights.weightPc  ShowAdditionalParam=off  OutDataTypeStr=double
  Data Store Read : DataStoreRead  DataStoreName=weightsPc  IndexOptions=Index vector (dialog)  Indices=1  OutputSizes=1
  Data Store Read1 : DataStoreRead  DataStoreName=weightsWc  IndexOptions=Index vector (dialog)  Indices=1  OutputSizes=1
  Data Store Read2 : DataStoreRead  DataStoreName=weightsZc  IndexOptions=Index vector (dialog)  Indices=1  OutputSizes=1
  Data Store Read3 : DataStoreRead  DataStoreName=weightsWc  IndexOptions=Index vector (dialog)  Indices=1  OutputSizes=1
  Data Store Read4 : DataStoreRead  DataStoreName=weightsZc  IndexOptions=Index vector (dialog)  Indices=1  OutputSizes=1
  Data Store Read5 : DataStoreRead  DataStoreName=weightsPc  IndexOptions=Index vector (dialog)  Indices=1  OutputSizes=1
  Data Store Read6 : DataStoreRead  DataStoreName=weightsWc  IndexOptions=Index vector (dialog)  Indices=1  OutputSizes=1
  Data Store Read7 : DataStoreRead  DataStoreName=weightsZc  IndexOptions=Index vector (dialog)  Indices=1  OutputSizes=1
  Data Store Read8 : DataStoreRead  DataStoreName=weightsPc  IndexOptions=Index vector (dialog)  Indices=1  OutputSizes=1
  Data Store Write : DataStoreWrite  DataStoreName=weightsPc  IndexOptions=Index vector (dialog)  Indices=1  OutputSizes=1
  Data Store Write1 : DataStoreWrite  DataStoreName=weightsZc  IndexOptions=Index vector (dialog)  Indices=1  OutputSizes=1
  Data Store Write2 : DataStoreWrite  DataStoreName=weightsWc  IndexOptions=Index vector (dialog)  Indices=1  OutputSizes=1
  Demux : Demux  Outputs=3
  Mux : Mux  Inputs=3
  Mux1 : Mux  Inputs=3
  Mux2 : Mux  Inputs=3
  Red Neuronal B-spline : MATLAB Function  TreatAsAtomicUnit=on
  To Workspace : ToWorkspace  VariableName=BSplineNN_weights  SaveFormat=Timeseries  SampleTime=-1
  bspline_gpi_params : Scope  NumInputPorts=3
  weights_BSplineNN : Scope  NumInputPorts=3
  Wc : Outport
  Zc : Outport  Port=2
  Pc : Outport  Port=3
  wires:
  e_q/1 -> Red Neuronal B-spline/2(e_q)
  [Bspline_params] -> Red Neuronal B-spline/1(NN_Bspline_params)
  Red Neuronal B-spline/1(Wc) -> bspline_gpi_params/1, Wc/1
  Red Neuronal B-spline/2(Zc) -> bspline_gpi_params/2, Zc/1
  Red Neuronal B-spline/3(Pc) -> bspline_gpi_params/3, Pc/1
  Constant3/1 -> [Bspline_params]
  Data Store Read1/1 -> Bus Creator/1  "weightsWc"
  Data Store Read5/1 -> Bus Creator/3  "weightsPc"
  Bus Creator/1 -> To Workspace/1
  Data Store Read4/1 -> Bus Creator/2  "weightsZc"
  Red Neuronal B-spline/4(newweightsWc) -> Data Store Write2/1
  Red Neuronal B-spline/5(newweightsZc) -> Data Store Write1/1
  Red Neuronal B-spline/6(newweightsPc) -> Data Store Write/1
  Data Store Read3/1 -> Red Neuronal B-spline/6(weightsWc)
  Data Store Read2/1 -> Red Neuronal B-spline/7(weightsZc)
  Data Store Read/1 -> Red Neuronal B-spline/8(weightsPc)
  Data Store Read6/1 -> weights_BSplineNN/1  "weightsWc"
  Data Store Read7/1 -> weights_BSplineNN/2  "weightsZc"
  Data Store Read8/1 -> weights_BSplineNN/3  "weightsPc"
  Mux1/1 -> Red Neuronal B-spline/4(e_py)
  Mux2/1 -> Red Neuronal B-spline/5(e_pz)
  Demux/3 -> Mux2/3, Mux2/2, Mux2/1
  e_p/1 -> Demux/1
  Demux/1 -> Mux/3, Mux/1, Mux/2
  Mux/1 -> Red Neuronal B-spline/3(e_px)
  Demux/2 -> Mux1/1, Mux1/3, Mux1/2

== system controlGPI_pos_3dof_conMI/ControladorGPI + NN/Red neuronal/Constants ==
  Action Port : ActionPort  ActionPortLabel=else
  Constant : Constant  Value=Wc
  Constant1 : Constant  Value=Zc
  Constant2 : Constant  Value=Pc
  Scope1 : Scope  NumInputPorts=3
  Wc : Outport
  Zc : Outport  Port=2
  Pc : Outport  Port=3
  wires:
  Constant/1 -> Wc/1, Scope1/1
  Constant2/1 -> Scope1/3, Pc/1
  Constant1/1 -> Zc/1, Scope1/2

== system controlGPI_pos_3dof_conMI/ControladorGPI + NN/Red neuronal/RBF NNs ==
  e_q : Inport
  de_q : Inport  Port=2
  e_p : Inport  Port=3
  Action Port : ActionPort  ActionPortLabel=elseif(u1 == 2)
  Bus Creator : BusCreator  Inputs=3
  Constant5 : Constant  Value=NN_RBF_params.struct  OutDataTypeStr=Bus: NN_RBF_params_bus
  Data Store Memory : DataStoreMemory  DataStoreName=weightsWc  WriteAfterWriteMsg=warning  InitialValue=NN_RBF_params.weights.weightWc  ShowAdditionalParam=off  OutDataTypeStr=double
  Data Store Memory1 : DataStoreMemory  DataStoreName=weightsZc  WriteAfterWriteMsg=warning  InitialValue=NN_RBF_params.weights.weightZc  ShowAdditionalParam=off  OutDataTypeStr=double
  Data Store Memory2 : DataStoreMemory  DataStoreName=weightsPc  WriteAfterWriteMsg=warning  InitialValue=NN_RBF_params.weights.weightPc  ShowAdditionalParam=off  OutDataTypeStr=double
  Data Store Read : DataStoreRead  DataStoreName=weightsPc  IndexOptions=Index vector (dialog)  Indices=1  OutputSizes=1
  Data Store Read1 : DataStoreRead  DataStoreName=weightsZc  IndexOptions=Index vector (dialog)  Indices=1  OutputSizes=1
  Data Store Read2 : DataStoreRead  DataStoreName=weightsWc  IndexOptions=Index vector (dialog)  Indices=1  OutputSizes=1
  Data Store Read3 : DataStoreRead  DataStoreName=weightsWc  IndexOptions=Index vector (dialog)  Indices=1  OutputSizes=1
  Data Store Read4 : DataStoreRead  DataStoreName=weightsZc  IndexOptions=Index vector (dialog)  Indices=1  OutputSizes=1
  Data Store Read5 : DataStoreRead  DataStoreName=weightsPc  IndexOptions=Index vector (dialog)  Indices=1  OutputSizes=1
  Data Store Read6 : DataStoreRead  DataStoreName=weightsWc  IndexOptions=Index vector (dialog)  Indices=1  OutputSizes=1
  Data Store Read7 : DataStoreRead  DataStoreName=weightsZc  IndexOptions=Index vector (dialog)  Indices=1  OutputSizes=1
  Data Store Read8 : DataStoreRead  DataStoreName=weightsPc  IndexOptions=Index vector (dialog)  Indices=1  OutputSizes=1
  Data Store Write : DataStoreWrite  DataStoreName=weightsPc  IndexOptions=Index vector (dialog)  Indices=1  OutputSizes=1
  Data Store Write1 : DataStoreWrite  DataStoreName=weightsZc  IndexOptions=Index vector (dialog)  Indices=1  OutputSizes=1
  Data Store Write2 : DataStoreWrite  DataStoreName=weightsWc  IndexOptions=Index vector (dialog)  Indices=1  OutputSizes=1
  Demux : Demux  Outputs=3
  Mux : Mux  Inputs=3
  Mux1 : Mux  Inputs=3
  Mux2 : Mux  Inputs=3
  Red Neuronal RBF : MATLAB Function  TreatAsAtomicUnit=on
  To Workspace : ToWorkspace  VariableName=RBFNN_weights  SaveFormat=Timeseries  SampleTime=-1
  rbf_gpi_params : Scope  NumInputPorts=3
  weights_RBFNN : Scope  NumInputPorts=3
  Wc : Outport
  Zc : Outport  Port=2
  Pc : Outport  Port=3
  wires:
  [RBF_params] -> Red Neuronal RBF/1(NN_RBF_params)
  e_q/1 -> Red Neuronal RBF/2(e_q)
  Red Neuronal RBF/1(Wc) -> rbf_gpi_params/1, Wc/1
  Red Neuronal RBF/2(Zc) -> rbf_gpi_params/2, Zc/1
  Red Neuronal RBF/3(Pc) -> rbf_gpi_params/3, Pc/1
  Data Store Read/1 -> Red Neuronal RBF/8("weightsPc ")
  Data Store Read1/1 -> Red Neuronal RBF/7("weightsZc ")
  Data Store Read2/1 -> Red Neuronal RBF/6("weightsWc ")
  Data Store Read3/1 -> Bus Creator/1  "weightsWc"
  Data Store Read4/1 -> Bus Creator/2  "weightsZc"
  Data Store Read5/1 -> Bus Creator/3  "weightsPc"
  Bus Creator/1 -> To Workspace/1
  Red Neuronal RBF/6(weightsPc) -> Data Store Write/1
  Red Neuronal RBF/4(weightsWc) -> Data Store Write2/1
  Red Neuronal RBF/5(weightsZc) -> Data Store Write1/1
  Data Store Read6/1 -> weights_RBFNN/1  "weightsWc"
  Data Store Read7/1 -> weights_RBFNN/2  "weightsZc"
  Data Store Read8/1 -> weights_RBFNN/3  "weightsPc"
  Constant5/1 -> [RBF_params]
  e_p/1 -> Demux/1
  Mux/1 -> Red Neuronal RBF/3(e_px)
  Demux/1 -> Mux/3, Mux/1, Mux/2
  Demux/2 -> Mux1/1, Mux1/3, Mux1/2
  Mux1/1 -> Red Neuronal RBF/4(e_py)
  Demux/3 -> Mux2/3, Mux2/2, Mux2/1
  Mux2/1 -> Red Neuronal RBF/5(e_pz)

== system controlGPI_pos_3dof_conMI/Trayectoria de referencia/Inicializar posición de robot manipulador/2 to 3 (3) ==
  In1 : Inport
  In2 : Inport  Port=2
  Demux3 : Demux  Outputs=3
  Demux4 : Demux  Outputs=3
  Mux10 : Mux  Inputs=2
  Mux8 : Mux  Inputs=2
  Mux9 : Mux  Inputs=2
  1 : Outport
  2 : Outport  Port=2
  3 : Outport  Port=3
  wires:
  Demux4/3 -> Mux10/2
  Demux3/1 -> Mux8/1
  Demux3/2 -> Mux9/1
  Mux9/1 -> 2/1
  Demux4/2 -> Mux9/2
  Demux4/1 -> Mux8/2
  Demux3/3 -> Mux10/1
  Mux8/1 -> 1/1
  Mux10/1 -> 3/1
  In1/1 -> Demux3/1
  In2/1 -> Demux4/1

== system controlGPI_pos_3dof_conMI/Actuadores (Motores de inducción)/MI1 + PBC Torque Controller/Controlador PBC/2 a 2(1) ==
  In1 : Inport
  In2 : Inport  Port=2
  Demux1 : Demux  Outputs=2
  Demux2 : Demux  Outputs=2
  Mux : Mux  Inputs=2
  Mux1 : Mux  Inputs=2
  Out1 : Outport
  Out2 : Outport  Port=2
  wires:
  Demux2/1 -> Mux/2
  Mux/1 -> Out1/1
  In2/1 -> Demux2/1
  In1/1 -> Demux1/1
  Demux1/1 -> Mux/1
  Demux1/2 -> Mux1/1
  Mux1/1 -> Out2/1
  Demux2/2 -> Mux1/2

== system controlGPI_pos_3dof_conMI/Actuadores (Motores de inducción)/MI1 + PBC Torque Controller/Controlador PBC/Corrientes y Flujos deseados ==
  w_R : Inport
  psi_Rref : Inport  Port=2
  tau_Rref : Inport  Port=3
  psi_Rmagref : Inport  Port=4
  dpsi_Rmagref1 : Inport  Port=5
  Corrientes/Flujos deseados : MATLAB Function  TreatAsAtomicUnit=on
  i_Sref : Outport
  dpsi_Rref : Outport  Port=2
  wires:
  tau_Rref/1 -> Corrientes/Flujos deseados/4(tau_Rref)
  Corrientes/Flujos deseados/1(i_Sref) -> i_Sref/1
  psi_Rref/1 -> Corrientes/Flujos deseados/3(psi_Rref)
  w_R/1 -> Corrientes/Flujos deseados/2(w_R)
  Corrientes/Flujos deseados/2(dpsi_Rref) -> dpsi_Rref/1
  psi_Rmagref/1 -> Corrientes/Flujos deseados/5(psi_Rmagref)
  dpsi_Rmagref1/1 -> Corrientes/Flujos deseados/6(dpsi_Rmagref)
  [MI_motor_params] -> Corrientes/Flujos deseados/1(MI_motor_params)

== system controlGPI_pos_3dof_conMI/Actuadores (Motores de inducción)/MI1 + PBC Torque Controller/Controlador PBC/Ley de control ==
  i_Sref : Inport
  d_iSref : Inport  Port=2
  psi_Rref : Inport  Port=3
  w_R : Inport  Port=4
  e_iS : Inport  Port=5
  Bus Selector : BusSelector  OutputSignals=epsilon_KiS
  K_iS : MATLAB Function  TreatAsAtomicUnit=on
  Ley de control : MATLAB Function  TreatAsAtomicUnit=on
  Scope17 : Scope
  U_S : Outport
  wires:
  [K_iS] -> Ley de control/7(KI_s)
  d_iSref/1 -> Ley de control/3(d_iSref)
  psi_Rref/1 -> Ley de control/4(psi_Rref)
  i_Sref/1 -> Ley de control/2(i_Sref)
  Ley de control/1(U_S) -> U_S/1
  w_R/1 -> [w_R], Ley de control/5(w_R)
  e_iS/1 -> Ley de control/6(e_Is)
  Bus Selector/1 -> K_iS/3(epsilon)  "<epsilon_KiS>"
  K_iS/1(K_iS) -> Scope17/1, [K_iS]
  [w_R] -> K_iS/2(w_R)
  [MI_motor_params] -> Ley de control/1(MI_motor_params)
  [MI_motor_params] -> K_iS/1(MI_motor_params)
  [PBC_params] -> Bus Selector/1

== system controlGPI_pos_3dof_conMI/Actuadores (Motores de inducción)/MI1 + PBC Torque Controller/Controlador PBC/Rampa+Ret ==
  Demux : Demux  Tag=STV Demux  Outputs=1
      settings: DisplayOption=none
  FromWs : FromWorkspace  Tag=STV FromWs  VariableName=tuvar
      SigBuilderData=|
      | common.afterFinalStr = 'Extrapolate'
      | common.sampleTime = 0
      | dataSet.timeRange = [0 20]
      | dataSet.name = 'Group 1'
      | sbobj.Groups.Name = 'Group 1'
      | sbobj.Groups.Signals.Name = 'Signal 1'
      | sbobj.Groups.Signals.XData = [0 0.5 1 20]
      | sbobj.Groups.Signals.YData = [0 0 0.64 0.64]
      | sbobj.Groups.TimeRange = [0 20]
  Signal 1 : Outport  Tag=STV Outport
  wires:
  Demux/1 -> Signal 1/1
  FromWs/1 -> Demux/1

== system controlGPI_pos_3dof_conMI/Actuadores (Motores de inducción)/MI1 + PBC Torque Controller/Controlador PBC/derivada Corrientes deseadas ==
  psi_Rref : Inport
  dpsi_Rref : Inport  Port=2
  psi_Rmagref : Inport  Port=3
  dpsi_Rmagref : Inport  Port=4
  ddpsi_Rmagref : Inport  Port=5
  tau_Rref : Inport  Port=6
  dtau_Rref : Inport  Port=7
  Scope10 : Scope
  derivada Corrientes deseadas : MATLAB Function  TreatAsAtomicUnit=on
  d_iSref : Outport
  wires:
  dpsi_Rref/1 -> derivada Corrientes deseadas/3(dpsi_Rref)
  tau_Rref/1 -> derivada Corrientes deseadas/7(tau_Rref)
  dtau_Rref/1 -> derivada Corrientes deseadas/8(dtau_Rref)
  dpsi_Rmagref/1 -> derivada Corrientes deseadas/5(dpsi_Rmagref)
  derivada Corrientes deseadas/1(d_iSref) -> Scope10/1, d_iSref/1
  psi_Rmagref/1 -> derivada Corrientes deseadas/4(psi_Rmagref)
  psi_Rref/1 -> derivada Corrientes deseadas/2(psi_Rref)
  ddpsi_Rmagref/1 -> derivada Corrientes deseadas/6(ddpsi_Rmagref)
  [MI_motor_params] -> derivada Corrientes deseadas/1(MI_motor_params)

== system controlGPI_pos_3dof_conMI/Actuadores (Motores de inducción)/MI2 + PBC Torque Controller/Controlador PBC/2 a 2(1) ==
  In1 : Inport
  In2 : Inport  Port=2
  Demux1 : Demux  Outputs=2
  Demux2 : Demux  Outputs=2
  Mux : Mux  Inputs=2
  Mux1 : Mux  Inputs=2
  Out1 : Outport
  Out2 : Outport  Port=2
  wires:
  Demux2/1 -> Mux/2
  Mux/1 -> Out1/1
  In2/1 -> Demux2/1
  In1/1 -> Demux1/1
  Demux1/1 -> Mux/1
  Demux1/2 -> Mux1/1
  Mux1/1 -> Out2/1
  Demux2/2 -> Mux1/2

== system controlGPI_pos_3dof_conMI/Actuadores (Motores de inducción)/MI2 + PBC Torque Controller/Controlador PBC/Corrientes y Flujos deseados ==
  w_R : Inport
  psi_Rref : Inport  Port=2
  tau_Rref : Inport  Port=3
  psi_Rmagref : Inport  Port=4
  dpsi_Rmagref1 : Inport  Port=5
  Corrientes/Flujos deseados : MATLAB Function  TreatAsAtomicUnit=on
  i_Sref : Outport
  dpsi_Rref : Outport  Port=2
  wires:
  tau_Rref/1 -> Corrientes/Flujos deseados/4(tau_Rref)
  Corrientes/Flujos deseados/1(i_Sref) -> i_Sref/1
  psi_Rref/1 -> Corrientes/Flujos deseados/3(psi_Rref)
  w_R/1 -> Corrientes/Flujos deseados/2(w_R)
  Corrientes/Flujos deseados/2(dpsi_Rref) -> dpsi_Rref/1
  psi_Rmagref/1 -> Corrientes/Flujos deseados/5(psi_Rmagref)
  dpsi_Rmagref1/1 -> Corrientes/Flujos deseados/6(dpsi_Rmagref)
  [MI_motor_params] -> Corrientes/Flujos deseados/1(MI_motor_params)

== system controlGPI_pos_3dof_conMI/Actuadores (Motores de inducción)/MI2 + PBC Torque Controller/Controlador PBC/Ley de control ==
  i_Sref : Inport
  d_iSref : Inport  Port=2
  psi_Rref : Inport  Port=3
  w_R : Inport  Port=4
  e_iS : Inport  Port=5
  Bus Selector : BusSelector  OutputSignals=epsilon_KiS
  K_iS : MATLAB Function  TreatAsAtomicUnit=on
  Ley de control : MATLAB Function  TreatAsAtomicUnit=on
  Scope17 : Scope
  U_S : Outport
  wires:
  [K_iS] -> Ley de control/7(KI_s)
  d_iSref/1 -> Ley de control/3(d_iSref)
  psi_Rref/1 -> Ley de control/4(psi_Rref)
  i_Sref/1 -> Ley de control/2(i_Sref)
  Ley de control/1(U_S) -> U_S/1
  w_R/1 -> [w_R], Ley de control/5(w_R)
  e_iS/1 -> Ley de control/6(e_Is)
  Bus Selector/1 -> K_iS/3(epsilon)  "<epsilon_KiS>"
  K_iS/1(K_iS) -> Scope17/1, [K_iS]
  [w_R] -> K_iS/2(w_R)
  [MI_motor_params] -> Ley de control/1(MI_motor_params)
  [MI_motor_params] -> K_iS/1(MI_motor_params)
  [PBC_params] -> Bus Selector/1

== system controlGPI_pos_3dof_conMI/Actuadores (Motores de inducción)/MI2 + PBC Torque Controller/Controlador PBC/Rampa+Ret ==
  Demux : Demux  Tag=STV Demux  Outputs=1
      settings: DisplayOption=none
  FromWs : FromWorkspace  Tag=STV FromWs  VariableName=tuvar
      SigBuilderData=|
      | common.afterFinalStr = 'Extrapolate'
      | common.sampleTime = 0
      | dataSet.timeRange = [0 20]
      | dataSet.name = 'Group 1'
      | sbobj.Groups.Name = 'Group 1'
      | sbobj.Groups.Signals.Name = 'Signal 1'
      | sbobj.Groups.Signals.XData = [0 0.5 1 20]
      | sbobj.Groups.Signals.YData = [0 0 0.64 0.64]
      | sbobj.Groups.TimeRange = [0 20]
  Signal 1 : Outport  Tag=STV Outport
  wires:
  Demux/1 -> Signal 1/1
  FromWs/1 -> Demux/1

== system controlGPI_pos_3dof_conMI/Actuadores (Motores de inducción)/MI2 + PBC Torque Controller/Controlador PBC/derivada Corrientes deseadas ==
  psi_Rref : Inport
  dpsi_Rref : Inport  Port=2
  psi_Rmagref : Inport  Port=3
  dpsi_Rmagref : Inport  Port=4
  ddpsi_Rmagref : Inport  Port=5
  tau_Rref : Inport  Port=6
  dtau_Rref : Inport  Port=7
  Scope10 : Scope
  derivada Corrientes deseadas : MATLAB Function  TreatAsAtomicUnit=on
  d_iSref : Outport
  wires:
  dpsi_Rref/1 -> derivada Corrientes deseadas/3(dpsi_Rref)
  tau_Rref/1 -> derivada Corrientes deseadas/7(tau_Rref)
  dtau_Rref/1 -> derivada Corrientes deseadas/8(dtau_Rref)
  dpsi_Rmagref/1 -> derivada Corrientes deseadas/5(dpsi_Rmagref)
  derivada Corrientes deseadas/1(d_iSref) -> Scope10/1, d_iSref/1
  psi_Rmagref/1 -> derivada Corrientes deseadas/4(psi_Rmagref)
  psi_Rref/1 -> derivada Corrientes deseadas/2(psi_Rref)
  ddpsi_Rmagref/1 -> derivada Corrientes deseadas/6(ddpsi_Rmagref)
  [MI_motor_params] -> derivada Corrientes deseadas/1(MI_motor_params)

== system controlGPI_pos_3dof_conMI/Actuadores (Motores de inducción)/MI3 + PBC Torque Controller/Controlador PBC/2 a 2(1) ==
  In1 : Inport
  In2 : Inport  Port=2
  Demux1 : Demux  Outputs=2
  Demux2 : Demux  Outputs=2
  Mux : Mux  Inputs=2
  Mux1 : Mux  Inputs=2
  Out1 : Outport
  Out2 : Outport  Port=2
  wires:
  Demux2/1 -> Mux/2
  Mux/1 -> Out1/1
  In2/1 -> Demux2/1
  In1/1 -> Demux1/1
  Demux1/1 -> Mux/1
  Demux1/2 -> Mux1/1
  Mux1/1 -> Out2/1
  Demux2/2 -> Mux1/2

== system controlGPI_pos_3dof_conMI/Actuadores (Motores de inducción)/MI3 + PBC Torque Controller/Controlador PBC/Corrientes y Flujos deseados ==
  w_R : Inport
  psi_Rref : Inport  Port=2
  tau_Rref : Inport  Port=3
  psi_Rmagref : Inport  Port=4
  dpsi_Rmagref1 : Inport  Port=5
  Corrientes/Flujos deseados : MATLAB Function  TreatAsAtomicUnit=on
  i_Sref : Outport
  dpsi_Rref : Outport  Port=2
  wires:
  tau_Rref/1 -> Corrientes/Flujos deseados/4(tau_Rref)
  Corrientes/Flujos deseados/1(i_Sref) -> i_Sref/1
  psi_Rref/1 -> Corrientes/Flujos deseados/3(psi_Rref)
  w_R/1 -> Corrientes/Flujos deseados/2(w_R)
  Corrientes/Flujos deseados/2(dpsi_Rref) -> dpsi_Rref/1
  psi_Rmagref/1 -> Corrientes/Flujos deseados/5(psi_Rmagref)
  dpsi_Rmagref1/1 -> Corrientes/Flujos deseados/6(dpsi_Rmagref)
  [MI_motor_params] -> Corrientes/Flujos deseados/1(MI_motor_params)

== system controlGPI_pos_3dof_conMI/Actuadores (Motores de inducción)/MI3 + PBC Torque Controller/Controlador PBC/Ley de control ==
  i_Sref : Inport
  d_iSref : Inport  Port=2
  psi_Rref : Inport  Port=3
  w_R : Inport  Port=4
  e_iS : Inport  Port=5
  Bus Selector : BusSelector  OutputSignals=epsilon_KiS
  K_iS : MATLAB Function  TreatAsAtomicUnit=on
  Ley de control : MATLAB Function  TreatAsAtomicUnit=on
  Scope17 : Scope
  U_S : Outport
  wires:
  [K_iS] -> Ley de control/7(KI_s)
  d_iSref/1 -> Ley de control/3(d_iSref)
  psi_Rref/1 -> Ley de control/4(psi_Rref)
  i_Sref/1 -> Ley de control/2(i_Sref)
  Ley de control/1(U_S) -> U_S/1
  w_R/1 -> [w_R], Ley de control/5(w_R)
  e_iS/1 -> Ley de control/6(e_Is)
  Bus Selector/1 -> K_iS/3(epsilon)  "<epsilon_KiS>"
  K_iS/1(K_iS) -> Scope17/1, [K_iS]
  [w_R] -> K_iS/2(w_R)
  [MI_motor_params] -> Ley de control/1(MI_motor_params)
  [MI_motor_params] -> K_iS/1(MI_motor_params)
  [PBC_params] -> Bus Selector/1

== system controlGPI_pos_3dof_conMI/Actuadores (Motores de inducción)/MI3 + PBC Torque Controller/Controlador PBC/Rampa+Ret ==
  Demux : Demux  Tag=STV Demux  Outputs=1
      settings: DisplayOption=none
  FromWs : FromWorkspace  Tag=STV FromWs  VariableName=tuvar
      SigBuilderData=|
      | common.afterFinalStr = 'Extrapolate'
      | common.sampleTime = 0
      | dataSet.timeRange = [0 20]
      | dataSet.name = 'Group 1'
      | sbobj.Groups.Name = 'Group 1'
      | sbobj.Groups.Signals.Name = 'Signal 1'
      | sbobj.Groups.Signals.XData = [0 0.5 1 20]
      | sbobj.Groups.Signals.YData = [0 0 0.64 0.64]
      | sbobj.Groups.TimeRange = [0 20]
  Signal 1 : Outport  Tag=STV Outport
  wires:
  Demux/1 -> Signal 1/1
  FromWs/1 -> Demux/1

== system controlGPI_pos_3dof_conMI/Actuadores (Motores de inducción)/MI3 + PBC Torque Controller/Controlador PBC/derivada Corrientes deseadas ==
  psi_Rref : Inport
  dpsi_Rref : Inport  Port=2
  psi_Rmagref : Inport  Port=3
  dpsi_Rmagref : Inport  Port=4
  ddpsi_Rmagref : Inport  Port=5
  tau_Rref : Inport  Port=6
  dtau_Rref : Inport  Port=7
  Scope10 : Scope
  derivada Corrientes deseadas : MATLAB Function  TreatAsAtomicUnit=on
  d_iSref : Outport
  wires:
  dpsi_Rref/1 -> derivada Corrientes deseadas/3(dpsi_Rref)
  tau_Rref/1 -> derivada Corrientes deseadas/7(tau_Rref)
  dtau_Rref/1 -> derivada Corrientes deseadas/8(dtau_Rref)
  dpsi_Rmagref/1 -> derivada Corrientes deseadas/5(dpsi_Rmagref)
  derivada Corrientes deseadas/1(d_iSref) -> Scope10/1, d_iSref/1
  psi_Rmagref/1 -> derivada Corrientes deseadas/4(psi_Rmagref)
  psi_Rref/1 -> derivada Corrientes deseadas/2(psi_Rref)
  ddpsi_Rmagref/1 -> derivada Corrientes deseadas/6(ddpsi_Rmagref)
  [MI_motor_params] -> derivada Corrientes deseadas/1(MI_motor_params)

== matlab function controlGPI_pos_3dof_conMI/ControladorGPI + NN/Red neuronal/B-Spline NNs/Red Neuronal B-spline ==
  data: NN_Bspline_params input; e_q input size=[3,1]; Wc output size=[3,1]; Zc output size=[3,1]; Pc output size=[3,1]; e_px input size=[3,1]; e_py input size=[3,1]; e_pz input size=[3,1]; newweightsWc output; newweightsZc output; newweightsPc output; weightsWc input; weightsZc input; weightsPc input
function [Wc, Zc, Pc, newweightsWc, newweightsZc, newweightsPc]   = BSpline_NN(NN_Bspline_params,e_q,e_px,e_py,e_pz,weightsWc,weightsZc,weightsPc)

deltaWc = NN_Bspline_params.delta.deltaWc;
deltaZc = NN_Bspline_params.delta.deltaZc;
deltaPc = NN_Bspline_params.delta.deltaPc;

lambdaWc = NN_Bspline_params.lambda.lambdaWc;
lambdaZc = NN_Bspline_params.lambda.lambdaZc;
lambdaPc = NN_Bspline_params.lambda.lambdaPc;

if NN_Bspline_params.num_inputs == 1
    nn_inputs = e_q;
elseif NN_Bspline_params.num_inputs == 4
    nn_inputs = [e_q,e_px,e_py,e_pz];
else
    nn_inputs = e_q;
end

delta = [deltaWc;
         deltaZc;
         deltaPc];

lambda = cat(1,lambdaWc,lambdaZc,lambdaPc);
weights = cat(1,weightsWc,weightsZc,weightsPc);

[newparams,newweights] = NN_Bspline.Gradient_Descent(delta,weights,lambda,nn_inputs);

Wc = newparams(1,:)';
Zc = newparams(2,:)';
Pc = newparams(3,:)';

newweightsWc = newweights(1,:,:);
newweightsZc = newweights(2,:,:);
newweightsPc = newweights(3,:,:);

end

== matlab function controlGPI_pos_3dof_conMI/ControladorGPI + NN/Red neuronal/RBF NNs/Red Neuronal RBF ==
  data: NN_RBF_params input; e_q input size=[3,1]; Wc output size=[3,1]; Zc output size=[3,1]; Pc output size=[3,1]; e_px input size=[3,1]; e_py input size=[3,1]; e_pz input size=[3,1]; weightsWc output; weightsZc output; weightsPc output; weightsWc input; weightsZc input; weightsPc input
function [Wc, Zc, Pc, weightsWc, weightsZc, weightsPc] = RBF_NN(NN_RBF_params,e_q,e_px,e_py,e_pz, weightsWc, weightsZc, weightsPc)

%k = NN_RBF_params.rbf_params.k;
centers = NN_RBF_params.rbf_params.C';
radius = NN_RBF_params.rbf_params.sigma;

deltaWc = NN_RBF_params.delta.deltaWc;
deltaZc = NN_RBF_params.delta.deltaZc;
deltaPc = NN_RBF_params.delta.deltaPc;

if NN_RBF_params.num_inputs == 1
    NNRBF_inputs = e_q;
elseif NN_RBF_params.num_inputs == 4
    NNRBF_inputs = [e_q,e_px,e_py,e_pz];
else
    NNRBF_inputs = e_q;
end

delta = [deltaWc;
         deltaZc;
         deltaPc];

weights = cat(1,weightsWc,weightsZc,weightsPc);

[newparams,newweights] = NN_RBF.Gradient_Descent(delta,weights,centers,radius,NNRBF_inputs);

Wc = newparams(1,:)';
Zc = newparams(2,:)';
Pc = newparams(3,:)';

weightsWc = newweights(1,:,:);
weightsZc = newweights(2,:,:);
weightsPc = newweights(3,:,:);

end

== matlab function controlGPI_pos_3dof_conMI/q to xyz (robot)/q to xyz (referencia) ==
  data: p output size=[3,3]; robot_params input; q input size=[3,1]; dq input size=[3,1]; ddq input size=[3,1]; dp output size=[3,1]; ddp output size=[3,1]
function [p,dp,ddp] = fcn(robot_params,q,dq,ddq)

[p,dp,ddp] = robot_cin.cin_dir_3dof(robot_params,q,dq,ddq);

== matlab function controlGPI_pos_3dof_conMI/Trayectoria de referencia/xyz to q (referencia) ==
  data: robot_params input; q output size=[3,1]; r input size=[3,1]; dr input size=[3,1]; ddr input size=[3,1]; dq output size=[3,1]; ddq output size=[3,1]
function [q,dq,ddq] = fcn(robot_params,r,dr,ddr)

[q,dq,ddq] = robot_cin.cin_inv_3dof(robot_params,r,dr,ddr);
